simulink model "drive"  (R2017a)
settings: Solver=VariableStepAuto  StartTime=0.0  StopTime=10  FixedStep=Ts  RelTol=1e-3
values from neighbouring files (symbols this model uses):
  alpha = 0.6    [main.m]
  Ts = 0.001    [main.m]
undefined symbols (not defined in the file or in its folder): driver
settings Model: Creator=nirvana1289  LastModifiedBy=nirvana1289

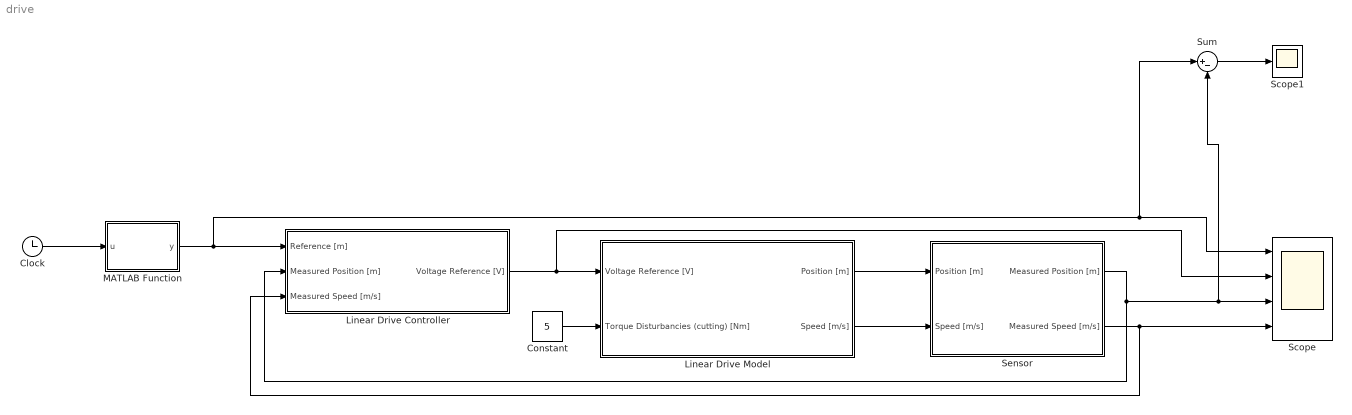
== system drive ==
  Clock : Clock
  Constant : Constant  Value=5
  Linear Drive Controller : Subsystem
  Linear Drive Model : Subsystem
  MATLAB Function : MATLAB Function  TreatAsAtomicUnit=on
  Scope : Scope  NumInputPorts=4
  Scope1 : Scope
  Sensor : Subsystem
  Sum : Sum  Inputs=|+-
  wires:
  Linear Drive Controller/1(Voltage Reference [V]) -> Scope/2, Linear Drive Model/1(Voltage Reference [V])
  Constant/1 -> Linear Drive Model/2(Torque Disturbancies (cutting) [Nm])
  MATLAB Function/1(y) -> Sum/1, Scope/1, Linear Drive Controller/1(Reference [m])
  Clock/1 -> MATLAB Function/1(u)
  Sensor/1(Measured Position [m]) -> Sum/2, Scope/3, Linear Drive Controller/2(Measured Position [m])
  Sensor/2(Measured Speed [m/s]) -> Scope/4, Linear Drive Controller/3(Measured Speed [m/s])
  Linear Drive Model/1(Position [m]) -> Sensor/1(Position [m])
  Linear Drive Model/2(Speed [m/s]) -> Sensor/2(Speed [m/s])
  Sum/1 -> Scope1/1

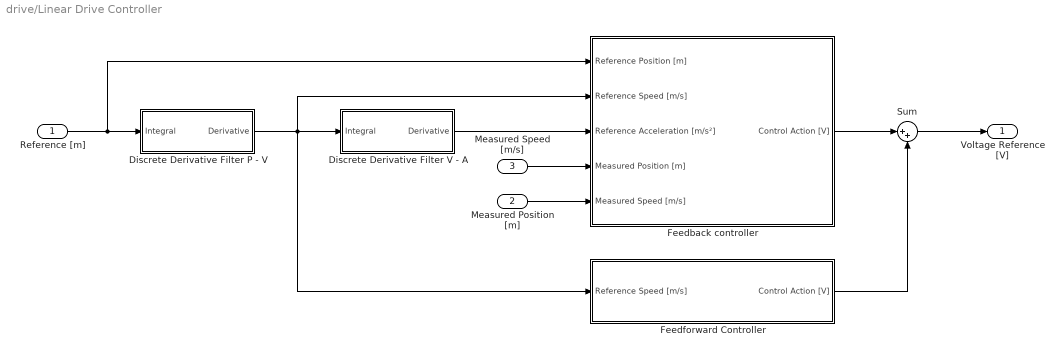
== system drive/Linear Drive Controller ==
  Reference [m] : Inport
  Measured Position [m] : Inport  Port=2
  Measured Speed [m/s] : Inport  Port=3
  Discrete Derivative Filter P - V : Subsystem
  Discrete Derivative Filter V - A : Subsystem
  Feedback controller : Subsystem
  Feedforward Controller : Subsystem
  Sum : Sum  Inputs=|++
  Voltage Reference [V] : Outport
  wires:
  Reference [m]/1 -> Feedback controller/1(Reference Position [m]), Discrete Derivative Filter P - V/1(Integral)
  Discrete Derivative Filter P - V/1(Derivative) -> Feedforward Controller/1(Reference Speed [m/s]), Discrete Derivative Filter V - A/1(Integral), Feedback controller/2(Reference Speed [m/s])
  Discrete Derivative Filter V - A/1(Derivative) -> Feedback controller/3(Reference Acceleration [m/s²])
  Measured Speed [m/s]/1 -> Feedback controller/4(Measured Position [m])
  Measured Position [m]/1 -> Feedback controller/5(Measured Speed [m/s])
  Feedback controller/1(Control Action [V]) -> Sum/1
  Feedforward Controller/1(Control Action [V]) -> Sum/2
  Sum/1 -> Voltage Reference [V]/1

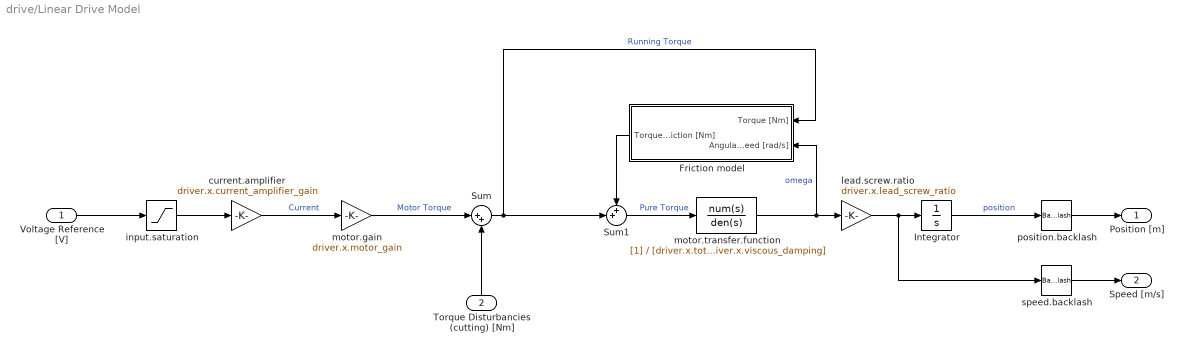
== system drive/Linear Drive Model ==
  Voltage Reference [V] : Inport
  Torque Disturbancies (cutting) [Nm] : Inport  Port=2
  Friction model : Subsystem
  Integrator : Integrator
  Sum : Sum  Inputs=|++
  Sum1 : Sum  Inputs=++|
  current.amplifier : Gain  Gain=driver.x.current_amplifier_gain
  input.saturation : Saturate  UpperLimit=driver.x.input_saturation  LowerLimit=-driver.x.input_saturation
  lead.screw.ratio : Gain  Gain=driver.x.lead_screw_ratio
  motor.gain : Gain  Gain=driver.x.motor_gain
  motor.transfer.function : TransferFcn  Denominator=[driver.x.total_reflected_inertia driver.x.viscous_damping]
  position.backlash : Backlash  BacklashWidth=driver.x.backlash_band
  speed.backlash : Backlash  BacklashWidth=driver.x.backlash_band
  Position [m] : Outport
  Speed [m/s] : Outport  Port=2
  wires:
  current.amplifier/1 -> motor.gain/1  "Current"
  motor.gain/1 -> Sum/1  "Motor Torque"
  Sum/1 -> Sum1/2, Friction model/1(Torque [Nm])  "Running Torque"
  motor.transfer.function/1 -> lead.screw.ratio/1, Friction model/2(Angular speed [rad/s])  "omega"
  Voltage Reference [V]/1 -> input.saturation/1
  lead.screw.ratio/1 -> speed.backlash/1, Integrator/1
  Torque Disturbancies (cutting) [Nm]/1 -> Sum/2
  input.saturation/1 -> current.amplifier/1
  Sum1/1 -> motor.transfer.function/1  "Pure Torque"
  Friction model/1(Torque friction [Nm]) -> Sum1/1
  Integrator/1 -> position.backlash/1  "position"
  position.backlash/1 -> Position [m]/1
  speed.backlash/1 -> Speed [m/s]/1

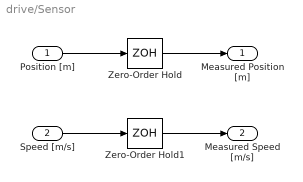
== system drive/Sensor ==
  Position [m] : Inport
  Speed [m/s] : Inport  Port=2
  Zero-Order Hold : ZeroOrderHold  SampleTime=Ts
  Zero-Order Hold1 : ZeroOrderHold  SampleTime=Ts
  Measured Position [m] : Outport
  Measured Speed [m/s] : Outport  Port=2
  wires:
  Position [m]/1 -> Zero-Order Hold/1
  Zero-Order Hold/1 -> Measured Position [m]/1
  Zero-Order Hold1/1 -> Measured Speed [m/s]/1
  Speed [m/s]/1 -> Zero-Order Hold1/1

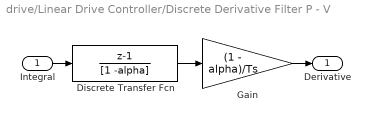
== system drive/Linear Drive Controller/Discrete Derivative Filter P - V ==
  Integral : Inport
  Discrete Transfer Fcn : DiscreteTransferFcn  Numerator=[1 -1]  Denominator=[1 -alpha]
  Gain : Gain  Gain=(1 - alpha)/Ts
  Derivative : Outport
  wires:
  Discrete Transfer Fcn/1 -> Gain/1
  Gain/1 -> Derivative/1
  Integral/1 -> Discrete Transfer Fcn/1

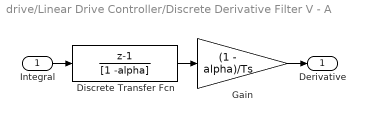
== system drive/Linear Drive Controller/Discrete Derivative Filter V - A ==
  Integral : Inport
  Discrete Transfer Fcn : DiscreteTransferFcn  Numerator=[1 -1]  Denominator=[1 -alpha]
  Gain : Gain  Gain=(1 - alpha)/Ts
  Derivative : Outport
  wires:
  Discrete Transfer Fcn/1 -> Gain/1
  Gain/1 -> Derivative/1
  Integral/1 -> Discrete Transfer Fcn/1

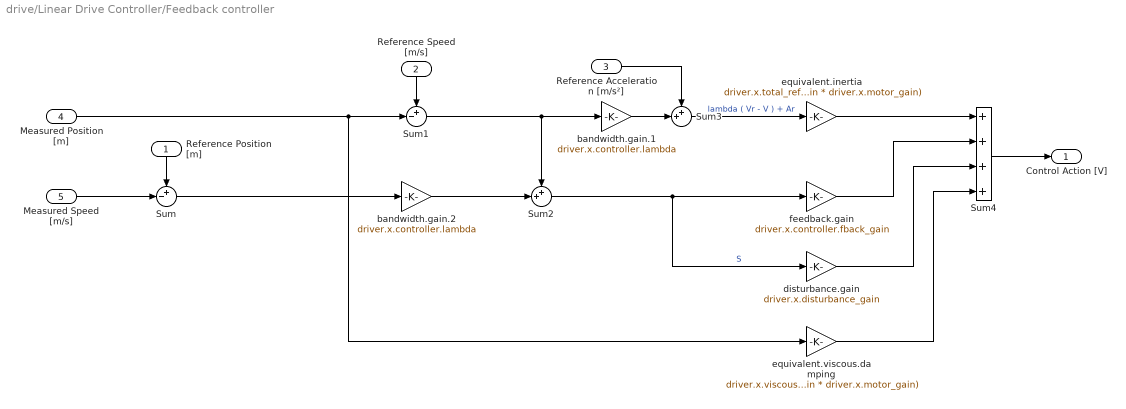
== system drive/Linear Drive Controller/Feedback controller ==
  Reference Position [m] : Inport
  Reference Speed [m/s] : Inport  Port=2
  Reference Acceleration [m/s²] : Inport  Port=3
  Measured Position [m] : Inport  Port=4
  Measured Speed [m/s] : Inport  Port=5
  Sum : Sum  Inputs=+-|
  Sum1 : Sum  Inputs=+-|
  Sum2 : Sum  Inputs=++|
  Sum3 : Sum  Inputs=++|
  Sum4 : Sum  Inputs=++++
  bandwidth.gain.1 : Gain  Gain=driver.x.controller.lambda
  bandwidth.gain.2 : Gain  Gain=driver.x.controller.lambda
  disturbance.gain : Gain  Gain=driver.x.disturbance_gain
  equivalent.inertia : Gain  Gain=driver.x.total_reflected_inertia/(driver.x.lead_screw_ratio * driver.x.current_amplifier_gain * driver.x.motor_gain)
  equivalent.viscous.damping : Gain  Gain=driver.x.viscous_damping/(driver.x.lead_screw_ratio * driver.x.current_amplifier_gain * driver.x.motor_gain)
  feedback.gain : Gain  Gain=driver.x.controller.fback_gain
  Control Action [V] : Outport
  wires:
  Sum3/1 -> equivalent.inertia/1  "lambda ( Vr - V ) + Ar"
  Reference Position [m]/1 -> Sum/1
  Reference Acceleration [m/s²]/1 -> Sum3/1
  Reference Speed [m/s]/1 -> Sum1/1
  disturbance.gain/1 -> Sum4/3
  bandwidth.gain.2/1 -> Sum2/2
  bandwidth.gain.1/1 -> Sum3/2
  equivalent.inertia/1 -> Sum4/1
  Measured Position [m]/1 -> equivalent.viscous.damping/1, Sum1/2
  Sum4/1 -> Control Action [V]/1
  equivalent.viscous.damping/1 -> Sum4/4
  Measured Speed [m/s]/1 -> Sum/2
  Sum/1 -> bandwidth.gain.2/1
  feedback.gain/1 -> Sum4/2
  Sum2/1 -> feedback.gain/1, disturbance.gain/1  "S"
  Sum1/1 -> bandwidth.gain.1/1, Sum2/1

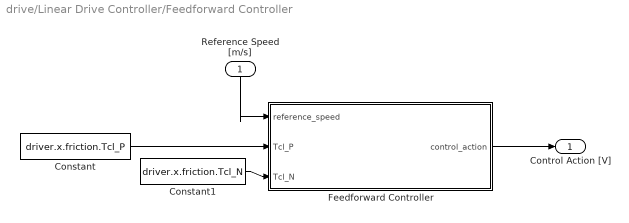
== system drive/Linear Drive Controller/Feedforward Controller ==
  Reference Speed [m/s] : Inport
  Constant : Constant  Value=driver.x.friction.Tcl_P
  Constant1 : Constant  Value=driver.x.friction.Tcl_N
  Feedforward Controller : MATLAB Function  TreatAsAtomicUnit=on
  Control Action [V] : Outport
  wires:
  Constant/1 -> Feedforward Controller/2(Tcl_P)
  Reference Speed [m/s]/1 -> Feedforward Controller/1(reference_speed)
  Constant1/1 -> Feedforward Controller/3(Tcl_N)
  Feedforward Controller/1(control_action) -> Control Action [V]/1

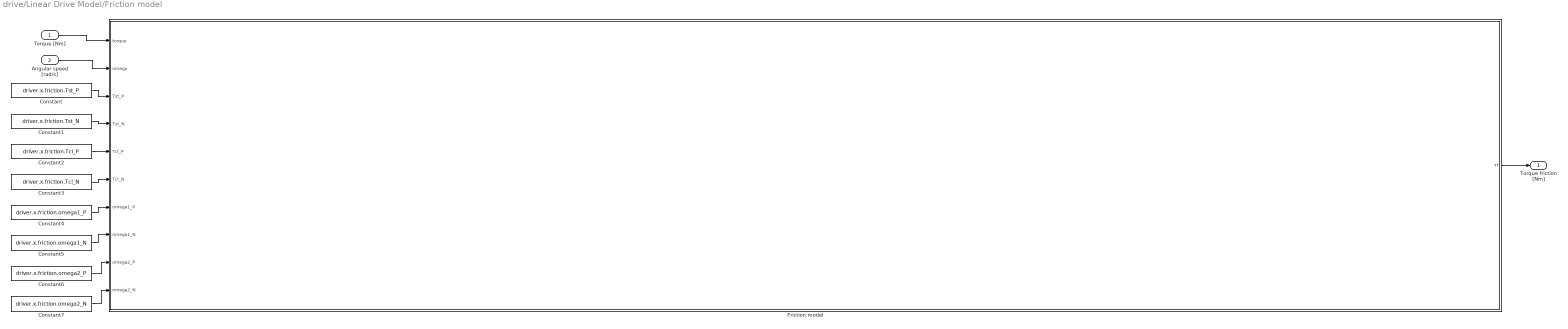
== system drive/Linear Drive Model/Friction model ==
  Torque [Nm] : Inport
  Angular speed [rad/s] : Inport  Port=2
  Constant : Constant  Value=driver.x.friction.Tst_P
  Constant1 : Constant  Value=driver.x.friction.Tst_N
  Constant2 : Constant  Value=driver.x.friction.Tcl_P
  Constant3 : Constant  Value=driver.x.friction.Tcl_N
  Constant4 : Constant  Value=driver.x.friction.omega1_P
  Constant5 : Constant  Value=driver.x.friction.omega1_N
  Constant6 : Constant  Value=driver.x.friction.omega2_P
  Constant7 : Constant  Value=driver.x.friction.omega2_N
  Friction model : MATLAB Function  TreatAsAtomicUnit=on
  Torque friction [Nm] : Outport
  wires:
  Friction model/1(Tf) -> Torque friction [Nm]/1
  Angular speed [rad/s]/1 -> Friction model/2(omega)
  Torque [Nm]/1 -> Friction model/1(torque)
  Constant/1 -> Friction model/3(Tst_P)
  Constant1/1 -> Friction model/4(Tst_N)
  Constant2/1 -> Friction model/5(Tcl_P)
  Constant3/1 -> Friction model/6(Tcl_N)
  Constant4/1 -> Friction model/7(omega1_P)
  Constant5/1 -> Friction model/8(omega1_N)
  Constant6/1 -> Friction model/9(omega2_P)
  Constant7/1 -> Friction model/10(omega2_N)

== matlab function drive/Linear Drive Controller/Feedforward Controller/Feedforward Controller ==
  data: reference_speed input; control_action output; Tcl_P input; Tcl_N input
function control_action = compensateFriction(reference_speed, Tcl_P, Tcl_N)
%#codegen
  if reference_speed > 0
      control_action = Tcl_P;
  elseif reference_speed < 0
      control_action = Tcl_N;
  else
      control_action = 0;
  end

== matlab function drive/Linear Drive Model/Friction model/Friction model ==
  data: torque input; Tf output; omega input; Tst_P input; Tst_N input; Tcl_P input; Tcl_N input; omega1_P input; omega1_N input; omega2_P input; omega2_N input
function Tf = fcn(torque, omega,  Tst_P, Tst_N, Tcl_P, Tcl_N, omega1_P, omega1_N, omega2_P, omega2_N)
%#codegen
  if omega > 0
     Tf = (Tst_P * exp(-omega/omega1_P) + Tcl_P * (1 - exp(-omega/omega2_P)));
  elseif omega < 0
     Tf = (Tst_N * exp(-omega/omega1_N) + Tcl_N * (1 - exp(-omega/omega2_N)));
  else
     if torque == 0
         Tf = 0.0;
     elseif torque > Tst_P
         Tf = Tst_P;
     elseif torque < Tst_N
         Tf = Tst_N; 
     else
         Tf = torque;
     end
  end

== matlab function drive/MATLAB Function ==
  data: u input; y output
function y = fcn(u)

y = -0.002 * u^3 + 0.03 * u^2;
